simulink model "sim_task_4"  (R2024a)
settings: Solver=FixedStepAuto  StartTime=0.0  StopTime=20.0  FixedStep=1e-3  RelTol=1e-3
settings Model: Creator=alexe  LastModifiedBy=alexe

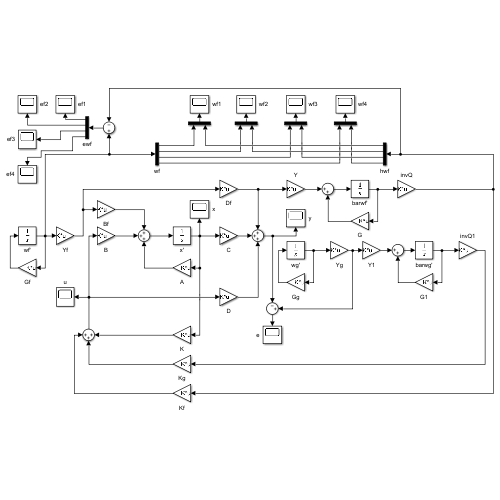
[thumbnail: Simulink's stored preview of the top-level diagram]
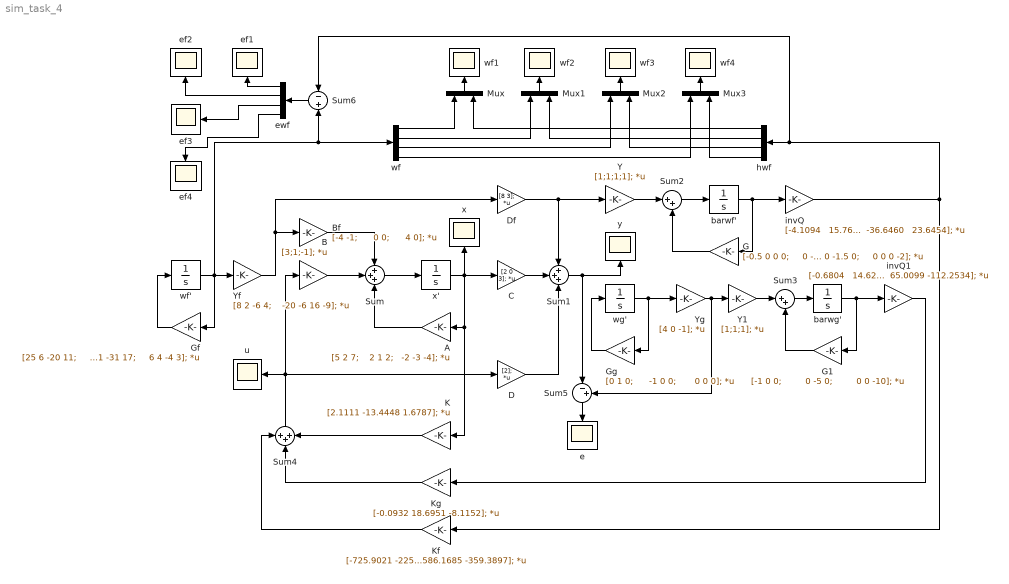
== system sim_task_4 ==
  A : Gain  Gain=|  Multiplication=Matrix(K*u)
      | [5 2 7;
      |    2 1 2;
      |   -2 -3 -4];
  B : Gain  Gain=[3;1;-1];  Multiplication=Matrix(K*u)
  Bf : Gain  Gain=|  Multiplication=Matrix(K*u)
      | [-4 -1;
      |      0 0;
      |      4 0];
  C : Gain  Gain=[2 0 3];  Multiplication=Matrix(K*u)
  D : Gain  Gain=[2];  Multiplication=Matrix(K*u)
  Df : Gain  Gain=[8 3];  Multiplication=Matrix(K*u)
  G : Gain  Gain=|  Multiplication=Matrix(K*u)
      | [-0.5 0 0 0;
      |     0 -1 0 0;
      |     0 0 -1.5 0;
      |     0 0 0 -2];
  G1 : Gain  Gain=|  Multiplication=Matrix(K*u)
      | [-1 0 0;
      |         0 -5 0;
      |         0 0 -10];
  Gf : Gain  Gain=|  Multiplication=Matrix(K*u)
      | [25 6 -20 11;
      |     14 3 -10 4;
      |     40 11 -31 17;
      |     6 4 -4 3];
  Gg : Gain  Gain=|  Multiplication=Matrix(K*u)
      | [0 1 0;
      |      -1 0 0;
      |       0 0 0];
  K : Gain  Gain=[2.1111 -13.4448 1.6787];  Multiplication=Matrix(K*u)
  Kf : Gain  Gain=[-725.9021 -225.1491 586.1685 -359.3897];  Multiplication=Matrix(K*u)
  Kg : Gain  Gain=[-0.0932 18.6951 -8.1152];  Multiplication=Matrix(K*u)
  Mux{,1..3} (4 alike) : Mux  Inputs=2
  Sum : Sum  Inputs=+++
  Sum1 : Sum  Inputs=+++
  Sum2 : Sum  Inputs=|++
  Sum3 : Sum  Inputs=|++
  Sum4 : Sum  Inputs=+++
  Sum5 : Sum  Inputs=|-+
  Sum6 : Sum  Inputs=-+
  Y : Gain  Gain=[1;1;1;1];  Multiplication=Matrix(K*u)
  Y1 : Gain  Gain=[1;1;1];  Multiplication=Matrix(K*u)
  Yf : Gain  Gain=|  Multiplication=Matrix(K*u)
      | [8 2 -6 4;
      |    -20 -6 16 -9];
  Yg : Gain  Gain=[4 0 -1];  Multiplication=Matrix(K*u)
  barwf' : Integrator  InitialCondition=[0;0;0;0];
  barwg' : Integrator  InitialCondition=[0;0;0];
  e : Scope
  ef{1..4} (4 alike) : Scope
  ewf : Demux
  hwf : Demux
  invQ : Gain  Gain=|  Multiplication=Matrix(K*u)
      | [-4.1094   15.7648  -19.2273    6.7770;
      |    -7.1320   34.6518  -56.9446   29.3341;
      |    -9.4484   43.5559  -68.5269   34.3983;
      |    -2.6486   17.2489  -36.6460   23.6454];
  invQ1 : Gain  Gain=|  Multiplication=Matrix(K*u)
      | [-0.6804   14.6291  -22.4543;
      |     0.2079  -17.8759   33.6724;
      |    -2.7766   65.0099 -112.2534];
  u : Scope
  wf : Demux
  wf' : Integrator  InitialCondition=[1;1;1;1];
  wf{1..4} (4 alike) : Scope
  wg' : Integrator  InitialCondition=[0;1;1];
  x : Scope
  x' : Integrator  InitialCondition=[0;0;0];
  y : Scope
  wires:
  x'/1 -> x/1, C/1, K/1, A/1
  Sum/1 -> x'/1
  A/1 -> Sum/3
  B/1 -> Sum/2
  Bf/1 -> Sum/1
  C/1 -> Sum1/2
  Df/1 -> Y/1, Sum1/1
  D/1 -> Sum1/3
  wf'/1 -> Sum6/2, wf/1, Yf/1, Gf/1
  Gf/1 -> wf'/1
  Yf/1 -> Bf/1, Df/1
  barwf'/1 -> invQ/1, G/1
  Sum2/1 -> barwf'/1
  Y/1 -> Sum2/1
  G/1 -> Sum2/2
  wg'/1 -> Yg/1, Gg/1
  Gg/1 -> wg'/1
  Yg/1 -> Sum5/2, Y1/1
  Y1/1 -> Sum3/1
  Sum3/1 -> barwg'/1
  G1/1 -> Sum3/2
  barwg'/1 -> invQ1/1, G1/1
  Sum4/1 -> u/1, D/1, B/1
  K/1 -> Sum4/3
  Kg/1 -> Sum4/2
  Kf/1 -> Sum4/1
  invQ1/1 -> Kg/1
  invQ/1 -> Sum6/1, hwf/1, Kf/1
  Sum1/1 -> Sum5/1, y/1
  Sum5/1 -> e/1
  wf/1 -> Mux/1
  hwf/1 -> Mux/2
  wf/2 -> Mux1/1
  hwf/2 -> Mux1/2
  wf/3 -> Mux2/1
  hwf/3 -> Mux2/2
  wf/4 -> Mux3/1
  hwf/4 -> Mux3/2
  Mux/1 -> wf1/1
  Mux1/1 -> wf2/1
  Mux2/1 -> wf3/1
  Mux3/1 -> wf4/1
  Sum6/1 -> ewf/1
  ewf/1 -> ef1/1
  ewf/2 -> ef2/1
  ewf/3 -> ef3/1
  ewf/4 -> ef4/1
